simulink model "F16_aero"  (Simulink 5.0)
settings: Solver=ode45  StartTime=0.0  StopTime=10.0  RelTol=1e-3
libraries: simulink x22
settings Model: Creator=bjax  LastModifiedBy=bjax  ExtModeAutoUpdateStatusClock=off  BooleanDataType=off

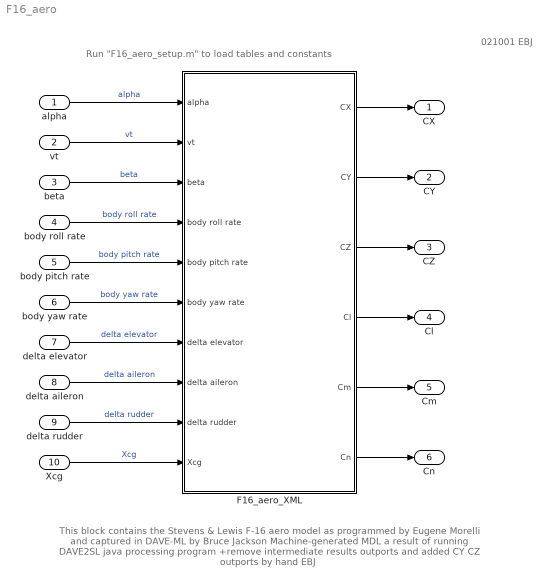
== system F16_aero ==
  note: This block contains the Stevens & Lewis F-16 aero model
      | as programmed by Eugene Morelli
      | and captured in DAVE-ML by Bruce Jackson
      | Machine-generated MDL a result of running DAVE2SL java processing program
      | +remove intermediate results outports and added CY CZ outports by hand EBJ
  note: 021001 EBJ
  note: Run "F16_aero_setup.m" to load tables and constants
  alpha : Inport
  vt : Inport  Port=2
  beta : Inport  Port=3
  body roll rate : Inport  Port=4
  body pitch rate : Inport  Port=5
  body yaw rate : Inport  Port=6
  delta elevator : Inport  Port=7
  delta aileron : Inport  Port=8
  delta rudder : Inport  Port=9
  Xcg : Inport  Port=10
  F16_aero_XML : Subsystem
  CX : Outport
  CY : Outport  Port=2
  CZ : Outport  Port=3
  Cl : Outport  Port=4
  Cm : Outport  Port=5
  Cn : Outport  Port=6
  wires:
  alpha/1 -> F16_aero_XML/1(alpha)  "alpha"
  F16_aero_XML/1(CX) -> CX/1
  F16_aero_XML/4(Cl) -> Cl/1
  F16_aero_XML/5(Cm) -> Cm/1
  F16_aero_XML/6(Cn) -> Cn/1
  vt/1 -> F16_aero_XML/2(vt)  "vt"
  beta/1 -> F16_aero_XML/3(beta)  "beta"
  body roll rate/1 -> F16_aero_XML/4(body roll rate)  "body roll rate"
  body pitch rate/1 -> F16_aero_XML/5(body pitch rate)  "body pitch rate"
  body yaw rate/1 -> F16_aero_XML/6(body yaw rate)  "body yaw rate"
  delta elevator/1 -> F16_aero_XML/7(delta elevator)  "delta elevator"
  delta aileron/1 -> F16_aero_XML/8(delta aileron)  "delta aileron"
  delta rudder/1 -> F16_aero_XML/9(delta rudder)  "delta rudder"
  Xcg/1 -> F16_aero_XML/10(Xcg)  "Xcg"
  F16_aero_XML/2(CY) -> CY/1
  F16_aero_XML/3(CZ) -> CZ/1

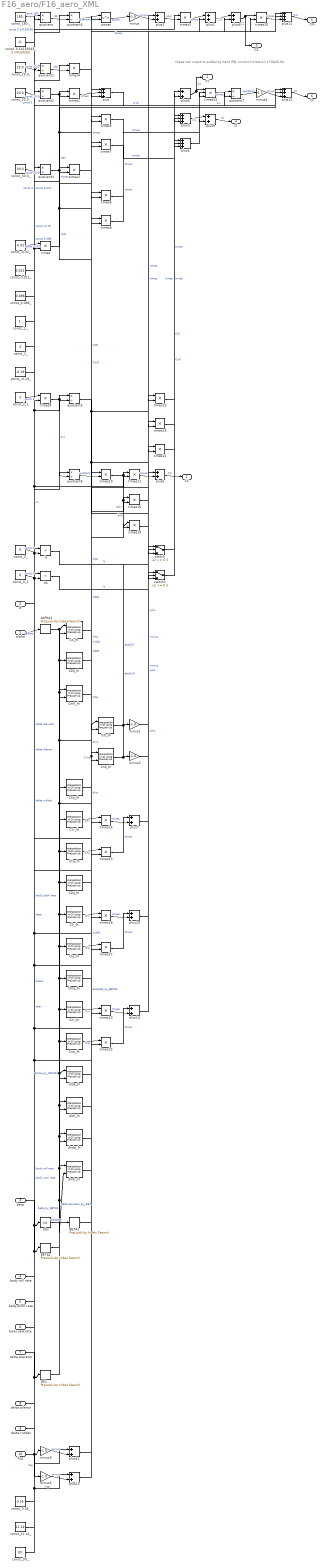
== system F16_aero/F16_aero_XML ==
  note: these two outports added by hand EBJ
      | current limitation of DAVE-ML
  alpha : Inport
  vt : Inport  Port=2
  beta : Inport  Port=3
  body roll rate : Inport  Port=4
  body pitch rate : Inport  Port=5
  body yaw rate : Inport  Port=6
  delta elevator : Inport  Port=7
  delta aileron : Inport  Port=8
  delta rudder : Inport  Port=9
  Xcg : Inport  Port=10
  ALPHA1 : simulink/Look-Up Tables/PreLook-Up Index Search  bpData=[-10.0, -5.0, 0.0, 5.0, 10.0, 15.0, 20.0, 25.0, 30.0, 35.0, 40.0, 45.0]  searchMode=Binary Search  cacheBpFlag=on  outputFlag=off  extrapMode=Linear Extrapolation  rangeErrorMode=None
  BETA1 : simulink/Look-Up Tables/PreLook-Up Index Search  bpData=[0.0, 5.0, 10.0, 15.0, 20.0, 25.0, 30.0]  searchMode=Binary Search  cacheBpFlag=on  outputFlag=off  extrapMode=Linear Extrapolation  rangeErrorMode=None
  BETA2 : simulink/Look-Up Tables/PreLook-Up Index Search  bpData=[-30.0, -20.0, -10.0, 0.0, 10.0, 20.0, 30.0]  searchMode=Binary Search  cacheBpFlag=on  outputFlag=off  extrapMode=Linear Extrapolation  rangeErrorMode=None
  CX_fn : simulink/Look-Up Tables/Interpolation (n-D) using PreLook-Up  numDimsPopupSelect=2  explicitNumDims=2  table=CX_table  interpMethod=Linear  extrapMethod=Linear  rangeErrorMode=None
  CXq_fn : simulink/Look-Up Tables/Interpolation (n-D) using PreLook-Up  numDimsPopupSelect=1  explicitNumDims=1  table=CXq_table  interpMethod=Linear  extrapMethod=Linear  rangeErrorMode=None
  CYp_fn : simulink/Look-Up Tables/Interpolation (n-D) using PreLook-Up  numDimsPopupSelect=1  explicitNumDims=1  table=CYp_table  interpMethod=Linear  extrapMethod=Linear  rangeErrorMode=None
  CYr_fn : simulink/Look-Up Tables/Interpolation (n-D) using PreLook-Up  numDimsPopupSelect=1  explicitNumDims=1  table=CYr_table  interpMethod=Linear  extrapMethod=Linear  rangeErrorMode=None
  CZ0_fn : simulink/Look-Up Tables/Interpolation (n-D) using PreLook-Up  numDimsPopupSelect=1  explicitNumDims=1  table=CZ0_table  interpMethod=Linear  extrapMethod=Linear  rangeErrorMode=None
  CZq_fn : simulink/Look-Up Tables/Interpolation (n-D) using PreLook-Up  numDimsPopupSelect=1  explicitNumDims=1  table=CZq_table  interpMethod=Linear  extrapMethod=Linear  rangeErrorMode=None
  Cl0_fn : simulink/Look-Up Tables/Interpolation (n-D) using PreLook-Up  numDimsPopupSelect=2  explicitNumDims=2  table=Cl0_table  interpMethod=Linear  extrapMethod=Linear  rangeErrorMode=None
  Clp_fn : simulink/Look-Up Tables/Interpolation (n-D) using PreLook-Up  numDimsPopupSelect=1  explicitNumDims=1  table=Clp_table  interpMethod=Linear  extrapMethod=Linear  rangeErrorMode=None
  Clr_fn : simulink/Look-Up Tables/Interpolation (n-D) using PreLook-Up  numDimsPopupSelect=1  explicitNumDims=1  table=Clr_table  interpMethod=Linear  extrapMethod=Linear  rangeErrorMode=None
  Cm0_fn : simulink/Look-Up Tables/Interpolation (n-D) using PreLook-Up  numDimsPopupSelect=2  explicitNumDims=2  table=Cm0_table  interpMethod=Linear  extrapMethod=Linear  rangeErrorMode=None
  Cmq_fn : simulink/Look-Up Tables/Interpolation (n-D) using PreLook-Up  numDimsPopupSelect=1  explicitNumDims=1  table=Cmq_table  interpMethod=Linear  extrapMethod=Linear  rangeErrorMode=None
  Cn0_fn : simulink/Look-Up Tables/Interpolation (n-D) using PreLook-Up  numDimsPopupSelect=2  explicitNumDims=2  table=Cn0_table  interpMethod=Linear  extrapMethod=Linear  rangeErrorMode=None
  Cnp_fn : simulink/Look-Up Tables/Interpolation (n-D) using PreLook-Up  numDimsPopupSelect=1  explicitNumDims=1  table=Cnp_table  interpMethod=Linear  extrapMethod=Linear  rangeErrorMode=None
  Cnr_fn : simulink/Look-Up Tables/Interpolation (n-D) using PreLook-Up  numDimsPopupSelect=1  explicitNumDims=1  table=Cnr_table  interpMethod=Linear  extrapMethod=Linear  rangeErrorMode=None
  DE1 : simulink/Look-Up Tables/PreLook-Up Index Search  bpData=[-24.0, -12.0, 0.0, 12.0, 24.0]  searchMode=Binary Search  cacheBpFlag=on  outputFlag=off  extrapMode=Linear Extrapolation  rangeErrorMode=None
  abs : Abs  SaturateOnIntegerOverflow=on
  const_-0.02_ : Constant  Value=-0.02
  const_-0.19_ : Constant  Value=-0.19
  const_0.021_ : Constant  Value=0.021
  const_0.086_ : Constant  Value=0.086
  const_0.35_ : Constant  Value=0.35
  const_0_ : Constant  Value=0
  const_0_1 : Constant  Value=0
  const_1._ : Constant  Value=1.
  const_11.32_ : Constant  Value=11.32
  const_180._ : Constant  Value=180.
  const_20.0_ : Constant  Value=20.0
  const_25.0_ : Constant  Value=25.0
  const_2_ : Constant  Value=2
  const_2_1 : Constant  Value=2
  const_3.14159265_ : Constant  Value=3.14159265
  const_30.0_ : Constant  Value=30.0
  const_30._ : Constant  Value=30.
  dlda_fn : simulink/Look-Up Tables/Interpolation (n-D) using PreLook-Up  numDimsPopupSelect=2  explicitNumDims=2  table=dlda_table  interpMethod=Linear  extrapMethod=Linear  rangeErrorMode=None
  dldr_fn : simulink/Look-Up Tables/Interpolation (n-D) using PreLook-Up  numDimsPopupSelect=2  explicitNumDims=2  table=dldr_table  interpMethod=Linear  extrapMethod=Linear  rangeErrorMode=None
  dnda_fn : simulink/Look-Up Tables/Interpolation (n-D) using PreLook-Up  numDimsPopupSelect=2  explicitNumDims=2  table=dnda_table  interpMethod=Linear  extrapMethod=Linear  rangeErrorMode=None
  dndr_fn : simulink/Look-Up Tables/Interpolation (n-D) using PreLook-Up  numDimsPopupSelect=2  explicitNumDims=2  table=dndr_table  interpMethod=Linear  extrapMethod=Linear  rangeErrorMode=None
  lt : RelationalOperator  Operator=<  InputSameDT=on
  lt1 : RelationalOperator  Operator=<  InputSameDT=on
  minus{,1..5} (6 alike) : Gain  Gain=-1.0  SaturateOnIntegerOverflow=on
  plus{,3..4,11,13} (5 alike) : Sum  Inputs=+++  SaturateOnIntegerOverflow=on  InputSameDT=on
  plus{1..2,5..10,12,14..15} (11 alike) : Sum  SaturateOnIntegerOverflow=on  InputSameDT=on
  power : Math  Operator=pow
  quotient{,1..7} (8 alike) : Product  Inputs=*/  SaturateOnIntegerOverflow=on  InputSameDT=on
  switch : Switch  Threshold=0.5  SaturateOnIntegerOverflow=on  InputSameDT=on
      settings: AttributesFormatString=Threshold = %<Threshold>
  switch1 : Switch  Threshold=0.5  SaturateOnIntegerOverflow=on  InputSameDT=on
      settings: AttributesFormatString=Threshold = %<Threshold>
  times{,1..23} (24 alike) : Product  SaturateOnIntegerOverflow=on  InputSameDT=on
  times24 : Product  Inputs=3  SaturateOnIntegerOverflow=on  InputSameDT=on
  CX : Outport
  CY : Outport  Port=2
  CZ : Outport  Port=3
  Cl : Outport  Port=4
  Cm : Outport  Port=5
  Cn : Outport  Port=6
  wires:
  vt/1 -> times9/2  "vt"
  alpha/1 -> ALPHA1/1  "alpha"
  beta/1 -> abs/1, BETA2/1, lt1/1, lt/1, times/2, quotient4/1  "beta"
  body roll rate/1 -> times13/2, times17/2, times22/2  "body roll rate"
  body pitch rate/1 -> quotient6/1  "body pitch rate"
  body yaw rate/1 -> times14/2, times18/2, times23/2  "body yaw rate"
  delta elevator/1 -> DE1/1, quotient1/1  "delta elevator"
  delta aileron/1 -> quotient2/1  "delta aileron"
  delta rudder/1 -> quotient3/1  "delta rudder"
  Xcg/1 -> minus3/1, minus5/1  "Xcg"
  quotient/1 -> quotient4/2  "rtd"
  const_180._/1 -> quotient/1  "const 180."
  const_3.14159265_/1 -> quotient/2  "const 3.14159265"
  const_0.35_/1 -> plus15/1, plus12/1  "xcgr"
  const_11.32_/1 -> times10/1, times24/3  "cbar"
  const_30._/1 -> quotient5/1, quotient7/2  "bspan"
  quotient1/1 -> times4/2  "del"
  const_25.0_/1 -> quotient1/2  "const 25.0"
  quotient2/1 -> times5/2, times7/2, times1/2  "dail"
  const_20.0_/1 -> quotient2/2  "const 20.0"
  quotient3/1 -> times6/2, times8/2, times2/2  "drdr"
  const_30.0_/1 -> quotient3/2  "const 30.0"
  CX_fn/1 -> plus5/1  "CX0"
  plus/1 -> plus6/1  "CY0"
  times/1 -> plus/1  "times"
  const_-0.02_/1 -> times/1  "const -0.02"
  times1/1 -> plus/2  "times"
  const_0.021_/1 -> times1/1  "const 0.021"
  times2/1 -> plus/3  "times"
  const_0.086_/1 -> times2/1  "const 0.086"
  CZ0_fn/1 -> times3/1  "CZ0"
  plus1/1 -> plus8/1  "CZ1"
  times3/1 -> plus1/1  "times"
  plus2/1 -> times3/2  "plus"
  const_1._/1 -> plus2/1  "const 1."
  minus/1 -> plus2/2  "minus"
  power/1 -> minus/1  "power"
  quotient4/1 -> power/1  "quotient"
  const_2_/1 -> power/2  "const 2"
  times4/1 -> plus1/2  "times"
  const_-0.19_/1 -> times4/1  "const -0.19"
  plus3/1 -> plus9/1  "Cl1"
  times5/1 -> plus3/2  "times"
  times6/1 -> plus3/3  "times"
  plus4/1 -> plus13/1  "Cn"
  times7/1 -> plus4/2  "times"
  times8/1 -> plus4/3  "times"
  times9/1 -> quotient6/2, quotient5/2  "tvt"
  const_2_1/1 -> times9/1  "const 2"
  quotient5/1 -> times12/1, times16/1, times21/1  "b2v"
  times10/1 -> times19/1, times15/1, times11/1  "cq2v"
  quotient6/1 -> times10/2  "quotient"
  abs/1 -> BETA1/1  "absbeta"
  Cl0_fn/1 -> switch/3, minus1/1  "absCl0"
  Cn0_fn/1 -> switch1/3, minus2/1  "absCn0"
  switch/1 -> plus3/1  "Cl0"
  minus1/1 -> switch/1  "minus"
  lt/1 -> switch/2  "lt"
  const_0_/1 -> lt/2  "const 0"
  Cm0_fn/1 -> plus11/1  "Cm0"
  switch1/1 -> plus4/1  "Cn0"
  minus2/1 -> switch1/1  "minus"
  lt1/1 -> switch1/2  "lt"
  const_0_1/1 -> lt1/2  "const 0"
  CXq_fn/1 -> times11/2  "CXq"
  CYr_fn/1 -> times14/1  "CYr"
  CYp_fn/1 -> times13/1  "CYp"
  CZq_fn/1 -> times15/2  "CZq"
  Clr_fn/1 -> times18/1  "Clr"
  Clp_fn/1 -> times17/1  "Clp"
  Cmq_fn/1 -> times19/2  "Cmq"
  Cnr_fn/1 -> times23/1  "Cnr"
  Cnp_fn/1 -> times22/1  "Cnp"
  dlda_fn/1 -> times5/1  "ClDA"
  dldr_fn/1 -> times6/1  "ClDR"
  dnda_fn/1 -> times7/1  "CnDA"
  dndr_fn/1 -> times8/1  "CnDR"
  plus5/1 -> CX/1  "CX"
  times11/1 -> plus5/2  "times"
  plus6/1 -> times24/1, CY/1  "CY"
  times12/1 -> plus6/2  "times"
  plus7/1 -> times12/2  "plus"
  times13/1 -> plus7/1  "times"
  times14/1 -> plus7/2  "times"
  plus8/1 -> times20/1, CZ/1  "CZ"
  times15/1 -> plus8/2  "times"
  plus9/1 -> Cl/1  "Cl"
  times16/1 -> plus9/2  "times"
  plus10/1 -> times16/2  "plus"
  times17/1 -> plus10/1  "times"
  times18/1 -> plus10/2  "times"
  plus11/1 -> Cm/1  "Cm"
  times19/1 -> plus11/2  "times"
  times20/1 -> plus11/3  "times"
  plus12/1 -> times20/2  "plus"
  minus3/1 -> plus12/2  "minus"
  plus13/1 -> Cn/1  "Cn"
  times21/1 -> plus13/2  "times"
  plus14/1 -> times21/2  "plus"
  times22/1 -> plus14/1  "times"
  times23/1 -> plus14/2  "times"
  minus4/1 -> plus13/3  "minus"
  quotient7/1 -> minus4/1  "quotient"
  times24/1 -> quotient7/1  "times"
  plus15/1 -> times24/2  "plus"
  minus5/1 -> plus15/2  "minus"
  DE1/1 -> CX_fn/1, Cm0_fn/1  "delta elevator_by_DE1"
  ALPHA1/1 -> Cl0_fn/2, Cn0_fn/2, dndr_fn/2, dnda_fn/2, dldr_fn/2, dlda_fn/2, Cnp_fn/1, Cnr_fn/1, Cmq_fn/1, Clp_fn/1, Clr_fn/1, CZq_fn/1, CYp_fn/1, CYr_fn/1, CXq_fn/1, Cm0_fn/2, CZ0_fn/1, CX_fn/2  "alpha_by_ALPHA1"
  BETA1/1 -> Cl0_fn/1, Cn0_fn/1  "absbeta_by_BETA1"
  BETA2/1 -> dlda_fn/1, dldr_fn/1, dnda_fn/1, dndr_fn/1  "beta_by_BETA2"
